simulink model "EasyModel"  (R2021a)
settings: Solver=FixedStepAuto  StartTime=0.0  StopTime=Inf  FixedStep=Ts  RelTol=1e-3
values from neighbouring files (symbols this model uses):
  Dir0 = [0;0]    [Preload.m]    (also in ResetFcn.m)
  flightplan = [2      0,   0;               150,   0, -60;               350,   0, -40;               zeros(18,3)]    [Preload.m]    (also in ResetFcn.m)
  obstacles = [1,     0,   0,  0;               0,     0,   0,  0 ... (first row only)    [Preload.m]    (also in ResetFcn.m)
  r0 = [0; 0; -50]    [Preload.m]    (also in ResetFcn.m)
libraries: rllib x1
settings Model: Creator=chitoshitamaoki  LastModifiedBy=chitoshitamaoki

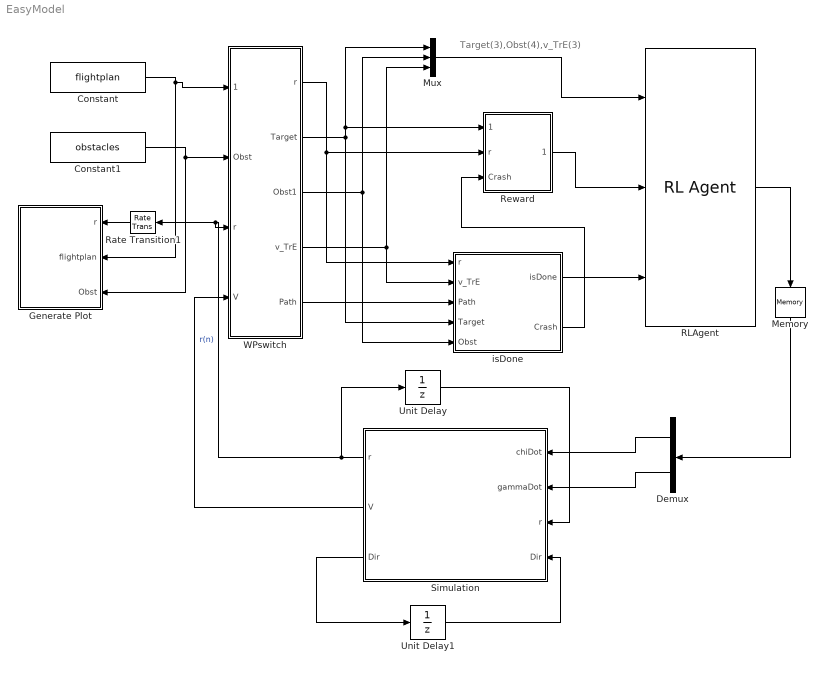
== system EasyModel ==
  note: Target(3),Obst(4),v_TrE(3)
  Constant : Constant  Value=flightplan
  Constant1 : Constant  Value=obstacles
  Demux : Demux  Outputs=2
  Generate Plot : MATLAB Function  TreatAsAtomicUnit=on
  Memory : Memory
  Mux : Mux  Inputs=3
  RLAgent : rllib/RL Agent  Agent=agent  ExternalActionAsInput=off  ProvideCumRwd=off  TreatAsDirectFeedthrough=on
  Rate Transition1 : RateTransition  OutPortSampleTimeOpt=Inherit  OutPortSampleTime=0.5
  Reward : MATLAB Function  TreatAsAtomicUnit=on
  Simulation : MATLAB Function  TreatAsAtomicUnit=on
  Unit Delay : UnitDelay  InitialCondition=r0  SampleTime=-1  HasFrameUpgradeWarning=on
  Unit Delay1 : UnitDelay  InitialCondition=Dir0  SampleTime=-1  HasFrameUpgradeWarning=on
  WPswitch : MATLAB Function  TreatAsAtomicUnit=on
  isDone : MATLAB Function  TreatAsAtomicUnit=on
  wires:
  Reward/1(Reward) -> RLAgent/2
  Mux/1 -> RLAgent/1
  WPswitch/2(Target) -> Mux/1, Reward/1(Target), isDone/4(Target)
  WPswitch/3(Obst1) -> Mux/2, isDone/5(Obst)
  WPswitch/4(v_TrE) -> Mux/3, isDone/2(v_TrE)
  WPswitch/1(r) -> isDone/1(r), Reward/2(r)
  WPswitch/5(Path) -> isDone/3(Path)
  Constant/1 -> WPswitch/1(flightplan), Generate Plot/2(flightplan)
  Constant1/1 -> WPswitch/2(Obst), Generate Plot/3(Obst)
  Rate Transition1/1 -> Generate Plot/1(r)
  Demux/2 -> Simulation/2(gammaDot)
  Demux/1 -> Simulation/1(chiDot)
  Unit Delay/1 -> Simulation/3("r ")
  Unit Delay1/1 -> Simulation/4("Dir ")
  Simulation/3(Dir) -> Unit Delay1/1
  Simulation/1(r) -> Rate Transition1/1, WPswitch/3("r "), Unit Delay/1  "r(n)"
  Simulation/2(V) -> WPswitch/4(V)
  RLAgent/1 -> Memory/1
  Memory/1 -> Demux/1
  isDone/2(Crash) -> Reward/3(Crash)
  isDone/1(isDone) -> RLAgent/3

== matlab function EasyModel/Generate Plot ==
  data: r input; flightplan input; Obst input
function fcn(r, flightplan, Obst)
%% Visualisierung
% coder.extrinsic('plot')
coder.extrinsic('animatedline')
coder.extrinsic('addpoints')
coder.extrinsic('get_param')
coder.extrinsic('delete')

persistent fig 
persistent handlePos
    
if isempty(fig)
    
    close all
    fig = figure('Name','State Monitor','WindowStyle','docked');
    
    
    wp_count = flightplan(1,1);
    ind = 2:(wp_count+1);
    plot3(flightplan(ind,2),...
          flightplan(ind,1),...
         -flightplan(ind,3),'k+');
    hold on
    
    %visualisation of WP
    N = 20;
    thetavec = linspace(0,pi,N);
    phivec = linspace(0,2*pi,2*N);
    [th, ph] = meshgrid(thetavec,phivec);
    R = ones(size(th));

    for i=2:(length(ind)+1)
    cx = flightplan(i,2);
    cy = flightplan(i,1);
    cz = flightplan(i,3);
    ro = 20;%must correspond to the value in WPswitch

    X = R.*sin(th).*cos(ph);
    Y = R.*sin(th).*sin(ph);
    Z = R.*cos(th);
     if norm(r-[cx;cy;cz])<ro
       surf(ro*X+cx,ro*Y+cy,ro*Z-cz,'EdgeColor','none','FaceColor','r','FaceAlpha',1);
     else
       surf(ro*X+cx,ro*Y+cy,ro*Z-cz,'EdgeColor','none','FaceColor','g','FaceAlpha',1);
     end
    end
    
    %visualisation of obstacles
    N = 20;
    thetavec = linspace(0,pi,N);
    phivec = linspace(0,2*pi,2*N);
    [th, ph] = meshgrid(thetavec,phivec);
    R = ones(size(th));

    for i=2:(length(ind)+1)
    cx = Obst(i,2);
    cy = Obst(i,1);
    cz = Obst(i,3);
    ro = Obst(i,4);

    X = R.*sin(th).*cos(ph);
    Y = R.*sin(th).*sin(ph);
    Z = R.*cos(th);
    if norm(r-[cx;cy;cz])<ro
       surf(ro*X+cx,ro*Y+cy,ro*Z-cz,'EdgeColor','none','FaceColor','y','FaceAlpha',1);
     else
       surf(ro*X+cx,ro*Y+cy,ro*Z-cz,'EdgeColor','none','FaceColor',[0.2 0.2 0.2],'FaceAlpha',1);
     end
    %surf(ro*X+cx,ro*Y+cy,ro*Z-cz,'EdgeColor','none','FaceColor',[0.2 0.2 0.2],'FaceAlpha',1);
    end
    
   
    ind = [2:(wp_count+1),2];
    hold on
    
    plot3(flightplan(ind,2),...
          flightplan(ind,1),...
         -flightplan(ind,3),'k--');
    handlePos = animatedline(0,0,0,'Color','r','LineWidth',1.5);
%     xlim([min(controller.flightplan(2:(wp_count+1),2))-50,max(controller.flightplan(2:(wp_count+1),2))+50]);
%     ylim([min(controller.flightplan(2:(wp_count+1),1))-50,max(controller.flightplan(2:(wp_count+1),1))+50]);
%     zlim([0,max(-controller.flightplan(2:(wp_count+1),3))+10]);
    xlabel('East [m]');
    ylabel('North [m]');
    zlabel('Height [m]');
    
    
    
    view(-30,45);%///////////////////
    %hText = text(0,0,'0');
    grid on;
    
end

addpoints(handlePos,r(2),r(1),-r(3));
%hText.String = "Speed:" + num2str(norm(VK)) + "m/s";
daspect([1 1 1])

drawnow limitrate

end

== matlab function EasyModel/Simulation ==
  data: chiDot input; r output; gammaDot input; V output; r input; Dir input; Dir output
function [r,V,Dir] = fcn(chiDot,gammaDot, r, Dir)

Ts = 0.01;
VK = 25;


Dir = Dir + [chiDot;gammaDot]*Ts;%[chi,gamma] Bahnwinkel von FZ in E-Ko.


V = zeros(3,1);
V = VK*[cos(Dir(2))*cos(Dir(1));%Absoluter Geschwindigkeitvektor in E-Ko.
        cos(Dir(2))*sin(Dir(1));
        -sin(Dir(2))       ];
    
 
r = r + V*Ts;%[X,Y,Z] in E-Ko.

if r(3)>0
    V = zeros(3,1);
end

end

== matlab function EasyModel/isDone ==
  data: r input; v_TrE input; Path input; Target input; isDone output; Obst input; Crash output
function [isDone,Crash] = isDone(r,v_TrE,Path,Target,Obst)

persistent steps
    if isempty(steps)
        steps = 1;
    end
    steps = steps+1;
if steps>20 && norm(v_TrE) <= 1
    isDone = true;
    Crash = 0;
    
    
elseif norm(Obst(1:3))<Obst(4)
    isDone = true;
    Crash = 1;
    
    
elseif r(1) < norm(Path)
     if sqrt(r(2)^2+r(3)^2)>100 %The gap to the fligt lane
        isDone = true;
        Crash = 0;
        
     else
        isDone =false;
        Crash = 0;
        
     end
elseif r(1) > norm(Path)
     if norm(Target)>100  %The gap to the currentWP
        isDone = true;
        Crash = 0;
        
     else
        isDone = false;
        Crash = 0;
        
     end


elseif steps>200%This must correspond to Tf. Cuz Tf is no avairable Parameter for this isDone funciton, you have to input it manually.
    isDone = true;
    Crash = 0;
    
else
    isDone = false;
    Crash = 0;
    
end

end

== matlab function EasyModel/WPswitch ==
  data: flightplan input; Obst input; r output; r input; Target output; Obst1 output; v_TrE output; Path output; V input
function [r, Target, Obst1, v_TrE, Path] = WPswitch(flightplan, Obst, r, V)
%% Assign constants
persistent CurrentWP_ID PreviousWP;

wp_count = flightplan(1,1);
WayPoints = flightplan(2:(wp_count+1),:)';
 
Obst = Obst(2:(wp_count+1),:)';

if (isempty(CurrentWP_ID))
    CurrentWP_ID = 1;
    %WPID = 1;
    PreviousWP = WayPoints(:,1);
end

CurrentWP = WayPoints(:,CurrentWP_ID);
%% WP switch

%radius = norm(CurrentWP - PreviousWP)/8;
if norm(r-CurrentWP) < 20 %if changed, change it in State Monitor too!!!
    CurrentWP_ID = CurrentWP_ID + 1;
    
    while CurrentWP_ID > 4
        CurrentWP_ID = CurrentWP_ID - 4;
    end
    
    if CurrentWP_ID > wp_count
   CurrentWP_ID = CurrentWP_ID - 1;
   end
    PreviousWP = CurrentWP;

end


%WPID = CurrentWP_ID;


%% Coordinate Transformation
Path = CurrentWP - PreviousWP;

%PathLength = single(zeros(1,1));
%PathLength = norm(Path);


chi0 = atan2(Path(2), Path(1));
gamma0 = atan2(-Path(3), sqrt(Path(1)^2+Path(2)^2));

TrE = [cos(gamma0)*cos(chi0), cos(gamma0)*sin(chi0), -sin(gamma0);
       -sin(chi0)           , cos(chi0)            , 0           ;
       sin(gamma0)*cos(chi0), sin(gamma0)*sin(chi0), cos(gamma0)];

r = TrE*(r - PreviousWP);

v_TrE = zeros(3,1);
v_TrE = TrE*V;

Target = zeros(3,1);

Target = TrE*(CurrentWP - PreviousWP);
Target = Target - r;%relative positions to WPs


Obst = Obst(:,2);
ObstNew = [Obst(1);Obst(2);Obst(3)];
ObstNew = TrE*(ObstNew - PreviousWP) - r;
Obst1 = zeros(4,1);
Obst1 = [ObstNew;Obst(4)];%relative position to obstacles

%No Transformation
%Target = CurrentWP - r;


end

== matlab function EasyModel/Reward ==
  data: Target input; r input; Reward output; Crash input
function Reward = Reward(Target, r, Crash)

CloserBonus = 20*exp(-0.00005*norm(Target)^2)-0.0001*Target(1)^2+10;



persistent Steps
if (isempty(Steps))
    Steps = 0;
end


if norm(Target)<20 && Steps ==0
    WPBonus = 1000;
    Steps = Steps +1;
elseif Steps > 0
    WPBonus = 1000;
    Steps = Steps +1;
else
    WPBonus = 0;
end



if Steps>29
    Steps = 0;
end

CrashPenalty = Crash * (-500);


GapToPath = 10*exp(-0.00005*norm([r(2);r(3)])^2)-10;


Reward = WPBonus + CrashPenalty + CloserBonus + GapToPath;


                     
end
